simulink model "EE5106_CA2_Pro4"  (R2021b)
settings: Solver=VariableStepAuto  StartTime=0.0  StopTime=10  RelTol=1e-3
settings Model: Creator=txx-rog  LastModifiedBy=txx-rog

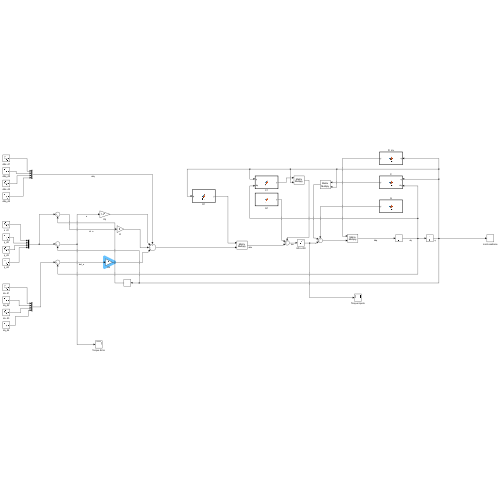
[thumbnail: Simulink's stored preview of the top-level diagram]
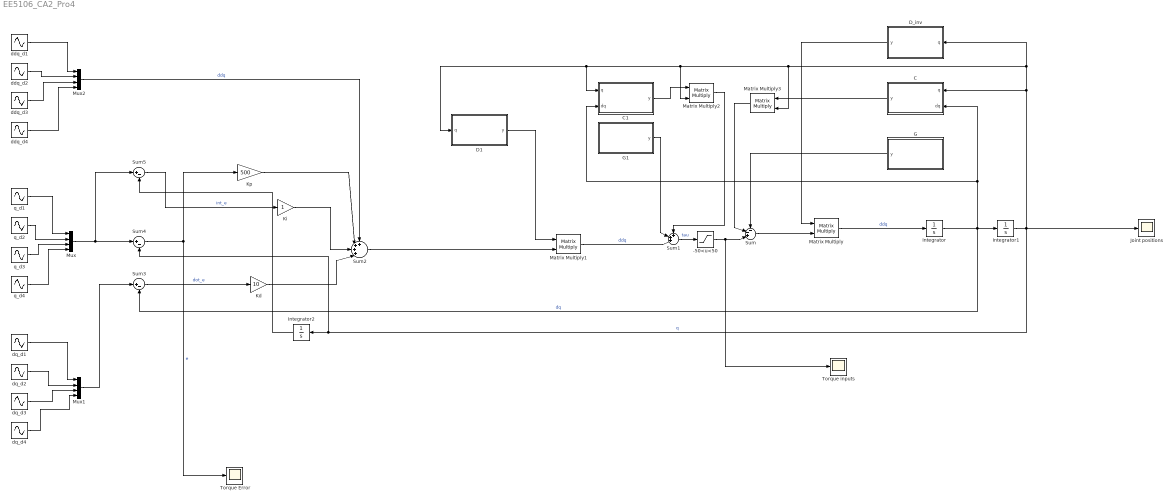
== system EE5106_CA2_Pro4 ==
  -50<u<50 : Saturate  UpperLimit=50  LowerLimit=-50
  C : MATLAB Function  TreatAsAtomicUnit=on
  C1 : MATLAB Function  TreatAsAtomicUnit=on
  D1 : MATLAB Function  TreatAsAtomicUnit=on
  D_inv : MATLAB Function  TreatAsAtomicUnit=on
  G : MATLAB Function  TreatAsAtomicUnit=on
  G1 : MATLAB Function  TreatAsAtomicUnit=on
  Integrator : Integrator
  Integrator1 : Integrator
  Integrator2 : Integrator
  Joint positions : Scope
  Kd : Gain  Gain=10
  Ki : Gain
  Kp : Gain  Gain=500
  Matrix Multiply{,1..3} (4 alike) : Product  Multiplication=Matrix(*)
  Mux : Mux
  Mux1 : Mux
  Mux2 : Mux
  Sum : Sum  Inputs=--+|
  Sum1 : Sum  Inputs=+++|
  Sum2 : Sum  Inputs=++++|
  Sum3 : Sum  Inputs=|+-
  Sum4 : Sum  Inputs=|+-
  Sum5 : Sum  Inputs=|+-
  Torque Error : Scope
  Torque inputs : Scope
  ddq_d1 : Sin  Amplitude=-0.5  SampleTime=0
  ddq_d2 : Sin  Amplitude=-0.2  SampleTime=0
  ddq_d3 : Sin  Amplitude=0.3  Frequency=2  Phase=-pi/2  SampleTime=0
  ddq_d4 : Sin  Amplitude=-0.4  SampleTime=0
  dq_d1 : Sin  Amplitude=-0.5  Phase=-pi/2  SampleTime=0
  dq_d2 : Sin  Amplitude=-0.2  Phase=-pi/2  SampleTime=0
  dq_d3 : Sin  Amplitude=-0.3  SampleTime=0
  dq_d4 : Sin  Amplitude=-0.4  Phase=-pi/2  SampleTime=0
  q_d1 : Sin  Amplitude=0.5  SampleTime=0
  q_d2 : Sin  Amplitude=0.2  SampleTime=0
  q_d3 : Sin  Amplitude=-0.3  Phase=-pi/2  SampleTime=0
  q_d4 : Sin  Amplitude=0.4  SampleTime=0
  wires:
  D_inv/1(y) -> Matrix Multiply/1
  Sum/1 -> Matrix Multiply/2
  G/1(y) -> Sum/1
  Matrix Multiply/1 -> Integrator/1  "ddq"
  Integrator/1 -> Sum3/2, C/2(dq), C1/2(dq), Integrator1/1  "dq"
  G1/1(y) -> Sum1/2
  Sum1/1 -> -50<u<50/1  "tau"
  D1/1(y) -> Matrix Multiply1/1
  Matrix Multiply1/1 -> Sum1/3  "ddq"
  Sum2/1 -> Matrix Multiply1/2
  dq_d2/1 -> Mux1/2
  dq_d3/1 -> Mux1/3
  dq_d4/1 -> Mux1/4
  ddq_d3/1 -> Mux2/3
  ddq_d2/1 -> Mux2/2
  ddq_d4/1 -> Mux2/4
  Kp/1 -> Sum2/2
  Ki/1 -> Sum2/3
  Kd/1 -> Sum2/4
  Integrator2/1 -> Sum5/2
  Mux1/1 -> Sum3/1
  Sum3/1 -> Kd/1  "dot_e"
  Mux/1 -> Sum4/1, Sum5/1
  q_d3/1 -> Mux/3
  q_d2/1 -> Mux/2
  q_d4/1 -> Mux/4
  Sum4/1 -> Torque Error/1, Kp/1  "e"
  Sum5/1 -> Ki/1  "int_e"
  Integrator1/1 -> Joint positions/1, C/1(q), Matrix Multiply3/2, D1/1(q), C1/1(q), Matrix Multiply2/2, D_inv/1(q), Sum4/2, Integrator2/1  "q"
  Mux2/1 -> Sum2/1  "ddq"
  Matrix Multiply2/1 -> Sum1/1
  Matrix Multiply3/1 -> Sum/2
  C1/1(y) -> Matrix Multiply2/1
  C/1(y) -> Matrix Multiply3/1
  ddq_d1/1 -> Mux2/1
  q_d1/1 -> Mux/1
  dq_d1/1 -> Mux1/1
  -50<u<50/1 -> Torque inputs/1, Sum/3

== matlab function EE5106_CA2_Pro4/C ==
  data: y output size=[4 4]; q input size=[4 1]; dq input size=[4 1]
function y  = fcn(q, dq)
 
C=zeros(4,4);
C(2,2) = - dq(4)*(0.12*sin(q(3)+q(4)) + 0.12*sin(q(4))) - dq(3)*(0.12*sin(q(3)+q(4)) + 0.704*sin(q(3)));
C(2,3) = - dq(4)*(0.12*sin(q(3)+q(4)) + 0.2*sin(q(4))) - dq(3)*(0.12*sin(q(3)+q(4)) + 0.96*sin(q(3))) - dq(2)*(0.12*sin(q(3)+q(4)) + 0.704*sin(q(3)));
C(2,4) = - dq(4)*(0.12*sin(q(3)+q(4)) + 0.12*sin(q(4))) - dq(3)*(0.12*sin(q(3)+q(4)) + 0.2*sin(q(4))) - dq(2)*(0.12*sin(q(3)+q(4))+ 0.12*sin(q(4))); 

C(3,2) = dq(2)*(0.12*sin(q(3)+q(4)) + 0.704*sin(q(3))) - dq(4)*0.2*sin(q(4));
C(3,3) = - dq(4)*0.12*sin(q(4));
C(3,4) = - dq(2)*0.2*sin(q(4))- dq(3)*0.12*sin(q(4)) - dq(4)*0.12*sin(q(4));
C(4,2) =  dq(2)*((0.12*sin(q(3)+q(4))) + 0.12*sin(q(4))) + dq(3)*0.2*sin(q(4));
C(4,3) =  dq(2)*0.2*sin(q(4)) + dq(3)*0.12*sin(q(4));

y = C;

== matlab function EE5106_CA2_Pro4/G ==
  data: y output
function y = fcn()

G=zeros(4,1);
mass = [1;1.2;1;0.6];
m1 = mass(1);
m2 = mass(2);
m3 = mass(3);
m4 = mass(4);
g = 9.8;



G(1) = (m1 + m2 + m3 + m4) * g;

y = G;

== matlab function EE5106_CA2_Pro4/D1 ==
  data: q input size=[4 1]; y output size=[4 4]
function y = fcn(q)

D=zeros(4,4); 

D(1,1) = 1;
D(2,2) = 1.408*cos(q(3))+0.24*cos(q(4))+0.24*cos(q(3)+q(4));
D(2,3) = 0.96*cos(q(3))+0.4*cos(q(4))+0.12*cos(q(3)+q(4))+1.1255;
D(2,4) = 0.12*cos(q(4))+0.12*cos(q(3)+q(4))+0.1125; 
D(3,2) = 0.96*cos(q(3))+0.4*cos(q(4))+0.12*cos(q(3)+q(4))+1.1255;
D(3,3) = 0.24*cos(q(4))+0.8695;
D(3,4) = 0.12*cos(q(4))+0.1125;
D(4,2) = 0.12*cos(q(4))+0.12*cos(q(3)+q(4))+0.1125;
D(4,3) = 0.12*cos(q(4))+0.1125;
D(4,4) = 0.1125;

y = D;

== matlab function EE5106_CA2_Pro4/C1 ==
  data: q input size=[4 1]; y output size=[4 4]; dq input size=[4 1]
function y = fcn(q,dq)
 
C=zeros(4,4);
C(2,2) = - dq(4)*(0.12*sin(q(3)+q(4)) + 0.12*sin(q(4))) - dq(3)*(0.12*sin(q(3)+q(4)) + 0.704*sin(q(3)));
C(2,3) = - dq(4)*(0.12*sin(q(3)+q(4)) + 0.2*sin(q(4))) - dq(3)*(0.12*sin(q(3)+q(4)) + 0.96*sin(q(3))) - dq(2)*(0.12*sin(q(3)+q(4)) + 0.704*sin(q(3)));
C(2,4) = - dq(4)*(0.12*sin(q(3)+q(4)) + 0.12*sin(q(4))) - dq(3)*(0.12*sin(q(3)+q(4)) + 0.2*sin(q(4))) - dq(2)*(0.12*sin(q(3)+q(4))+ 0.12*sin(q(4))); 

C(3,2) = dq(2)*(0.12*sin(q(3)+q(4)) + 0.704*sin(q(3))) - dq(4)*0.2*sin(q(4));
C(3,3) = - dq(4)*0.12*sin(q(4));
C(3,4) = - dq(2)*0.2*sin(q(4))- dq(3)*0.12*sin(q(4)) - dq(4)*0.12*sin(q(4));
C(4,2) =  dq(2)*((0.12*sin(q(3)+q(4))) + 0.12*sin(q(4))) + dq(3)*0.2*sin(q(4));
C(4,3) =  dq(2)*0.2*sin(q(4)) + dq(3)*0.12*sin(q(4));

y = C;

== matlab function EE5106_CA2_Pro4/G1 ==
  data: y output
function y = fcn()

G=zeros(4,1);
mass = [1;1.2;1;0.6];
m1 = mass(1);
m2 = mass(2);
m3 = mass(3);
m4 = mass(4);
g = 9.8;



G(1) = (m1 + m2 + m3 + m4) * g;

y = G;

== matlab function EE5106_CA2_Pro4/D_inv ==
  data: q input size=[4 1]; y output size=[4 4]
function y = fcn(q)

D=zeros(4,4); 

D(1,1) = 1;
D(2,2) = 1.408*cos(q(3))+0.24*cos(q(4))+0.24*cos(q(3)+q(4));
D(2,3) = 0.96*cos(q(3))+0.4*cos(q(4))+0.12*cos(q(3)+q(4))+1.1255;
D(2,4) = 0.12*cos(q(4))+0.12*cos(q(3)+q(4))+0.1125; 
D(3,2) = 0.96*cos(q(3))+0.4*cos(q(4))+0.12*cos(q(3)+q(4))+1.1255;
D(3,3) = 0.24*cos(q(4))+0.8695;
D(3,4) = 0.12*cos(q(4))+0.1125;
D(4,2) = 0.12*cos(q(4))+0.12*cos(q(3)+q(4))+0.1125;
D(4,3) = 0.12*cos(q(4))+0.1125;
D(4,4) = 0.1125;

y = inv(D);
